simulink model "fixpt_sl_product_mul4"  (Simulink 7.9)
settings: Solver=FixedStepDiscrete  StartTime=0.0  StopTime=0  FixedStep=1  RelTol=1e-3
settings Model: Creator=y_yama  LastModifiedBy=amatsumo
settings DataIOCC: SaveOutput=off  SignalLogging=off  SaveTime=off
settings OptimizationCC: BlockReduction=off  ConditionallyExecuteInputs=off  InlineParams=on  InlineInvariantSignals=on  ZeroExternalMemoryAtStartup=off  ZeroInternalMemoryAtStartup=off  InitFltsAndDblsToZero=on  NoFixptDivByZeroProtection=on  EfficientFloat2IntCast=on  OptimizeModelRefInitCode=on  LifeSpan=1
settings DebuggingCC: InheritedTsInSrcMsg=none  FcnCallInpInsideContextMsg=Use local settings  StrictBusMsg=Warning
settings HardwareCC: ProdHWDeviceType=ASIC/FPGA->ASIC/FPGA  TargetEndianess=LittleEndian  TargetHWDeviceType=MATLAB Host  ProdEqTarget=off
settings RTWCC: SystemTargetFile=ert.tlc  GenCodeOnly=on  TemplateMakefile=ert_default_tmf  Description=Real-Time Workshop Embedded Coder (no auto configuration)  GenerateReport=on  ProcessScript=ert_make_rtw_hook  IncludeHyperlinkInReport=on  LaunchReport=on
settings CodeAppCC: GenerateComments=off  IgnoreCustomStorageClasses=off  CustomSymbolStrGlobalVar=$N$M  SimulinkBlockComments=off
settings ERTTargetCC: CodeReplacementLibrary=ANSI_C  MultiwordLength=2048  GenerateSampleERTMain=on  IncludeMdlTerminateFcn=off  SuppressErrorStatus=on  SupportAbsoluteTime=off  SupportNonFinite=off  SupportComplex=off  PurelyIntegerCode=on  InlinedParameterPlacement=NonHierarchical  ERTCustomFileTemplate=example_file_process.tlc  ConvertIfToSwitch=off  SuppressUnreachableDefaultCases=off

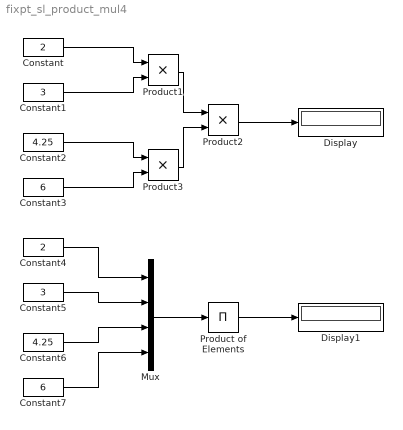
== system fixpt_sl_product_mul4 ==
  Constant : Constant  Value=2  OutDataTypeStr=fixdt(1,8,1)  SampleTime=-1
      settings: AttributesFormatString=DataType = %<OutDataTypeStr>
  Constant1 : Constant  Value=3  OutDataTypeStr=fixdt(1,8,1)  SampleTime=-1
      settings: AttributesFormatString=DataType = %<OutDataTypeStr>
  Constant2 : Constant  Value=4.25  OutDataTypeStr=fixdt(1,8,1)  SampleTime=-1
      settings: AttributesFormatString=DataType = %<OutDataTypeStr>
  Constant3 : Constant  Value=6  OutDataTypeStr=fixdt(1,8,1)  SampleTime=-1
      settings: AttributesFormatString=DataType = %<OutDataTypeStr>
  Constant4 : Constant  Value=2  OutDataTypeStr=fixdt(1,8,1)  SampleTime=-1
      settings: AttributesFormatString=DataType = %<OutDataTypeStr>
  Constant5 : Constant  Value=3  OutDataTypeStr=fixdt(1,8,1)  SampleTime=-1
      settings: AttributesFormatString=DataType = %<OutDataTypeStr>
  Constant6 : Constant  Value=4.25  OutDataTypeStr=fixdt(1,8,1)  SampleTime=-1
      settings: AttributesFormatString=DataType = %<OutDataTypeStr>
  Constant7 : Constant  Value=6  OutDataTypeStr=fixdt(1,8,1)  SampleTime=-1
      settings: AttributesFormatString=DataType = %<OutDataTypeStr>
  Display : Display
      settings: AttributesFormatString=Format = %<Format>
  Display1 : Display
      settings: AttributesFormatString=Format = %<Format>
  Mux : Mux
  Product of Elements : Product  Inputs=*  RndMeth=Nearest
  Product1 : Product  RndMeth=Nearest
  Product2 : Product  RndMeth=Nearest
  Product3 : Product  RndMeth=Nearest
  wires:
  Product2/1 -> Display/1
  Constant/1 -> Product1/1
  Constant1/1 -> Product1/2
  Constant2/1 -> Product3/1
  Constant3/1 -> Product3/2
  Mux/1 -> Product of Elements/1
  Product of Elements/1 -> Display1/1
  Constant4/1 -> Mux/1
  Constant5/1 -> Mux/2
  Constant6/1 -> Mux/3
  Constant7/1 -> Mux/4
  Product3/1 -> Product2/2
  Product1/1 -> Product2/1
